simulink model "test_mdl1"  (R2023a)
settings: Solver=VariableStepAuto  StartTime=0.0  StopTime=10.0  RelTol=1e-3
(part 4 of 8)

== system test_mdl1/VehicleCAN/GWM/Climate_Cntrl_Data_2_FD1 ==
  AutoStpHvacDelta_I_Est : Constant  Value=0
  CabnAmb_Te_Actl : Constant  Value=0
  ClimtThrmlLoad_No_Actl : Constant  Value=0
  HvacAir_Flw_Est : Constant  Value=0
  HvacBlwrFront_D_Stat : Constant  Value=0
  HvacRec_Pc_Est : Constant  Value=0
  HvacRemoteStrt_N_Rq : Constant  Value=0
  bus_creator : BusCreator  Inputs=7
  out_port : Outport
  wires:
  bus_creator/1 -> out_port/1  "test_mdl1"
  AutoStpHvacDelta_I_Est/1 -> bus_creator/1  "AutoStpHvacDelta_I_Est"
  CabnAmb_Te_Actl/1 -> bus_creator/2  "CabnAmb_Te_Actl"
  ClimtThrmlLoad_No_Actl/1 -> bus_creator/3  "ClimtThrmlLoad_No_Actl"
  HvacAir_Flw_Est/1 -> bus_creator/4  "HvacAir_Flw_Est"
  HvacBlwrFront_D_Stat/1 -> bus_creator/5  "HvacBlwrFront_D_Stat"
  HvacRec_Pc_Est/1 -> bus_creator/6  "HvacRec_Pc_Est"
  HvacRemoteStrt_N_Rq/1 -> bus_creator/7  "HvacRemoteStrt_N_Rq"

== system test_mdl1/VehicleCAN/GWM/Climate_Control_Data_FD1 ==
  AutoHoldSwtch_D_Stat : Constant  Value=0
  LpdbDfrstRearOn_B_Rq : Constant  Value=0
  LpdbHeatWiprPrk_B_Rq : Constant  Value=0
  LpdbPtc1_B_Rq : Constant  Value=0
  LpdbPtc2_B_Rq : Constant  Value=0
  LpdbPtc3_B_Rq : Constant  Value=0
  MirrorHeatOn_B_Rq : Constant  Value=0
  Outside_Air_Temp_Stat : Constant  Value=0
  Remote_Start_QuietMode : Constant  Value=0
  SteWhlHeat_D_Rq : Constant  Value=0
  bus_creator : BusCreator  Inputs=10
  out_port : Outport
  wires:
  bus_creator/1 -> out_port/1  "test_mdl1"
  AutoHoldSwtch_D_Stat/1 -> bus_creator/1  "AutoHoldSwtch_D_Stat"
  LpdbDfrstRearOn_B_Rq/1 -> bus_creator/2  "LpdbDfrstRearOn_B_Rq"
  LpdbHeatWiprPrk_B_Rq/1 -> bus_creator/3  "LpdbHeatWiprPrk_B_Rq"
  LpdbPtc1_B_Rq/1 -> bus_creator/4  "LpdbPtc1_B_Rq"
  LpdbPtc2_B_Rq/1 -> bus_creator/5  "LpdbPtc2_B_Rq"
  LpdbPtc3_B_Rq/1 -> bus_creator/6  "LpdbPtc3_B_Rq"
  MirrorHeatOn_B_Rq/1 -> bus_creator/7  "MirrorHeatOn_B_Rq"
  Outside_Air_Temp_Stat/1 -> bus_creator/8  "Outside_Air_Temp_Stat"
  Remote_Start_QuietMode/1 -> bus_creator/9  "Remote_Start_QuietMode"
  SteWhlHeat_D_Rq/1 -> bus_creator/10  "SteWhlHeat_D_Rq"

== system test_mdl1/VehicleCAN/GWM/Cluster_HEV_Data8_FD1 ==
  ConsAvgTrip_Fe_Dsply : Constant  Value=0
  DrvEffLvl_No_Stat : Constant  Value=0
  EngAirFilt_B_RqReset : Constant  Value=0
  GpsElMdeSel_B_Rq : Constant  Value=0
  LongTermReset_B_Rq : Constant  Value=0
  bus_creator : BusCreator  Inputs=5
  out_port : Outport
  wires:
  bus_creator/1 -> out_port/1  "test_mdl1"
  ConsAvgTrip_Fe_Dsply/1 -> bus_creator/1  "ConsAvgTrip_Fe_Dsply"
  DrvEffLvl_No_Stat/1 -> bus_creator/2  "DrvEffLvl_No_Stat"
  EngAirFilt_B_RqReset/1 -> bus_creator/3  "EngAirFilt_B_RqReset"
  GpsElMdeSel_B_Rq/1 -> bus_creator/4  "GpsElMdeSel_B_Rq"
  LongTermReset_B_Rq/1 -> bus_creator/5  "LongTermReset_B_Rq"

== system test_mdl1/VehicleCAN/GWM/Cluster_Info1_FD1 ==
  AccDeny_B_RqIpc : Constant  Value=0
  AccEnbl_B_RqDrv : Constant  Value=0
  BulbChkActv_B_Stat : Constant  Value=0
  DrvSlipCtlMde_B_Rq2 : Constant  Value=0
  DrvSlipCtlMde_D_Rq : Constant  Value=0
  EngIdlShutDown_B_RqDrv : Constant  Value=0
  EngOilLife_B_RqReset : Constant  Value=0
  HaDsplyCpblty_B_Stat : Constant  Value=0
  HsaMde_D_Rq : Constant  Value=0
  KeyTypeChngMykey_D_Rq : Constant  Value=0
  LscmbbStat_B_Actl : Constant  Value=0
  ManRgen_D_Rq : Constant  Value=0
  MetricActv_B_Actl : Constant  Value=0
  NtrlTowMdeEnbl_B_RqDrv : Constant  Value=0
  OdometerMasterValue : Constant  Value=0
  ParkDetect_Stat : Constant  Value=0
  Power_Liftgate_Mode_Cmd : Constant  Value=0
  ReducedGuard_D_Rq : Constant  Value=0
  TRAILER_BRAKE_CONFIG : Constant  Value=0
  TRLR_SWAY_CONFIG_CMD : Constant  Value=0
  TrlrBrkMde_D_Rq : Constant  Value=0
  bus_creator : BusCreator  Inputs=22
  ePRNDL_MODE : Constant  Value=0
  out_port : Outport
  wires:
  bus_creator/1 -> out_port/1  "test_mdl1"
  AccDeny_B_RqIpc/1 -> bus_creator/1  "AccDeny_B_RqIpc"
  AccEnbl_B_RqDrv/1 -> bus_creator/2  "AccEnbl_B_RqDrv"
  BulbChkActv_B_Stat/1 -> bus_creator/3  "BulbChkActv_B_Stat"
  DrvSlipCtlMde_B_Rq2/1 -> bus_creator/4  "DrvSlipCtlMde_B_Rq2"
  DrvSlipCtlMde_D_Rq/1 -> bus_creator/5  "DrvSlipCtlMde_D_Rq"
  EngIdlShutDown_B_RqDrv/1 -> bus_creator/6  "EngIdlShutDown_B_RqDrv"
  EngOilLife_B_RqReset/1 -> bus_creator/7  "EngOilLife_B_RqReset"
  HaDsplyCpblty_B_Stat/1 -> bus_creator/8  "HaDsplyCpblty_B_Stat"
  HsaMde_D_Rq/1 -> bus_creator/9  "HsaMde_D_Rq"
  KeyTypeChngMykey_D_Rq/1 -> bus_creator/10  "KeyTypeChngMykey_D_Rq"
  LscmbbStat_B_Actl/1 -> bus_creator/11  "LscmbbStat_B_Actl"
  ManRgen_D_Rq/1 -> bus_creator/12  "ManRgen_D_Rq"
  MetricActv_B_Actl/1 -> bus_creator/13  "MetricActv_B_Actl"
  NtrlTowMdeEnbl_B_RqDrv/1 -> bus_creator/14  "NtrlTowMdeEnbl_B_RqDrv"
  OdometerMasterValue/1 -> bus_creator/15  "OdometerMasterValue"
  ParkDetect_Stat/1 -> bus_creator/16  "ParkDetect_Stat"
  Power_Liftgate_Mode_Cmd/1 -> bus_creator/17  "Power_Liftgate_Mode_Cmd"
  ReducedGuard_D_Rq/1 -> bus_creator/18  "ReducedGuard_D_Rq"
  TRAILER_BRAKE_CONFIG/1 -> bus_creator/19  "TRAILER_BRAKE_CONFIG"
  TRLR_SWAY_CONFIG_CMD/1 -> bus_creator/20  "TRLR_SWAY_CONFIG_CMD"
  TrlrBrkMde_D_Rq/1 -> bus_creator/21  "TrlrBrkMde_D_Rq"
  ePRNDL_MODE/1 -> bus_creator/22  "ePRNDL_MODE"

== system test_mdl1/VehicleCAN/GWM/Cluster_Info_3_FD1 ==
  AutoRgen_D_Rq : Constant  Value=0
  DISPLAY_SPEED_OFFSET : Constant  Value=0
  DISPLAY_SPEED_SCALING : Constant  Value=0
  DrvSlipCtlMde_B_RqMyKey : Constant  Value=0
  FUEL_SENSOR_NUM : Constant  Value=0
  FuelLvlActvSide_No_Raw : Constant  Value=0
  FuelLvlPssvSide_No_Raw : Constant  Value=0
  FuelLvlWarn_D_Actl : Constant  Value=0
  FuelLvl_Pc_Dsply : Constant  Value=0
  FuelSecndActv_B_Actl : Constant  Value=0
  HILL_DESC_SW : Constant  Value=0
  OdoTripRx_B_Actl : Constant  Value=0
  Veh_V_CompLimMx : Constant  Value=0
  W2S_LAMP_OK : Constant  Value=0
  bus_creator : BusCreator  Inputs=14
  out_port : Outport
  wires:
  bus_creator/1 -> out_port/1  "test_mdl1"
  AutoRgen_D_Rq/1 -> bus_creator/1  "AutoRgen_D_Rq"
  DISPLAY_SPEED_OFFSET/1 -> bus_creator/2  "DISPLAY_SPEED_OFFSET"
  DISPLAY_SPEED_SCALING/1 -> bus_creator/3  "DISPLAY_SPEED_SCALING"
  DrvSlipCtlMde_B_RqMyKey/1 -> bus_creator/4  "DrvSlipCtlMde_B_RqMyKey"
  FUEL_SENSOR_NUM/1 -> bus_creator/5  "FUEL_SENSOR_NUM"
  FuelLvlActvSide_No_Raw/1 -> bus_creator/6  "FuelLvlActvSide_No_Raw"
  FuelLvlPssvSide_No_Raw/1 -> bus_creator/7  "FuelLvlPssvSide_No_Raw"
  FuelLvlWarn_D_Actl/1 -> bus_creator/8  "FuelLvlWarn_D_Actl"
  FuelLvl_Pc_Dsply/1 -> bus_creator/9  "FuelLvl_Pc_Dsply"
  FuelSecndActv_B_Actl/1 -> bus_creator/10  "FuelSecndActv_B_Actl"
  HILL_DESC_SW/1 -> bus_creator/11  "HILL_DESC_SW"
  OdoTripRx_B_Actl/1 -> bus_creator/12  "OdoTripRx_B_Actl"
  Veh_V_CompLimMx/1 -> bus_creator/13  "Veh_V_CompLimMx"
  W2S_LAMP_OK/1 -> bus_creator/14  "W2S_LAMP_OK"

== system test_mdl1/VehicleCAN/GWM/Cluster_Lighting_Rq_FD1 ==
  IsaOffst_D_Rq : Constant  Value=0
  SlMde_D_Rq : Constant  Value=0
  bus_creator : BusCreator  Inputs=2
  out_port : Outport
  wires:
  bus_creator/1 -> out_port/1  "test_mdl1"
  IsaOffst_D_Rq/1 -> bus_creator/1  "IsaOffst_D_Rq"
  SlMde_D_Rq/1 -> bus_creator/2  "SlMde_D_Rq"

== system test_mdl1/VehicleCAN/GWM/Compressor_Req_FD1 ==
  ClimtCool_D_Rq : Constant  Value=0
  ClimtHeat_D_Rq : Constant  Value=0
  ClimtPw_B_Rq : Constant  Value=0
  HvacAirCond_B_Rq : Constant  Value=0
  HvacEvap_Te_Actl : Constant  Value=0
  HvacEvap_Te_Offst : Constant  Value=0
  HvacEvap_Te_Rq : Constant  Value=0
  HvacHtrCore_Te_Rq : Constant  Value=0
  SnowPlowMde_B_Enbl : Constant  Value=0
  StopStrtDrvMde_B_RqBtn : Constant  Value=0
  bus_creator : BusCreator  Inputs=10
  out_port : Outport
  wires:
  bus_creator/1 -> out_port/1  "test_mdl1"
  ClimtCool_D_Rq/1 -> bus_creator/1  "ClimtCool_D_Rq"
  ClimtHeat_D_Rq/1 -> bus_creator/2  "ClimtHeat_D_Rq"
  ClimtPw_B_Rq/1 -> bus_creator/3  "ClimtPw_B_Rq"
  HvacAirCond_B_Rq/1 -> bus_creator/4  "HvacAirCond_B_Rq"
  HvacEvap_Te_Actl/1 -> bus_creator/5  "HvacEvap_Te_Actl"
  HvacEvap_Te_Offst/1 -> bus_creator/6  "HvacEvap_Te_Offst"
  HvacEvap_Te_Rq/1 -> bus_creator/7  "HvacEvap_Te_Rq"
  HvacHtrCore_Te_Rq/1 -> bus_creator/8  "HvacHtrCore_Te_Rq"
  SnowPlowMde_B_Enbl/1 -> bus_creator/9  "SnowPlowMde_B_Enbl"
  StopStrtDrvMde_B_RqBtn/1 -> bus_creator/10  "StopStrtDrvMde_B_RqBtn"

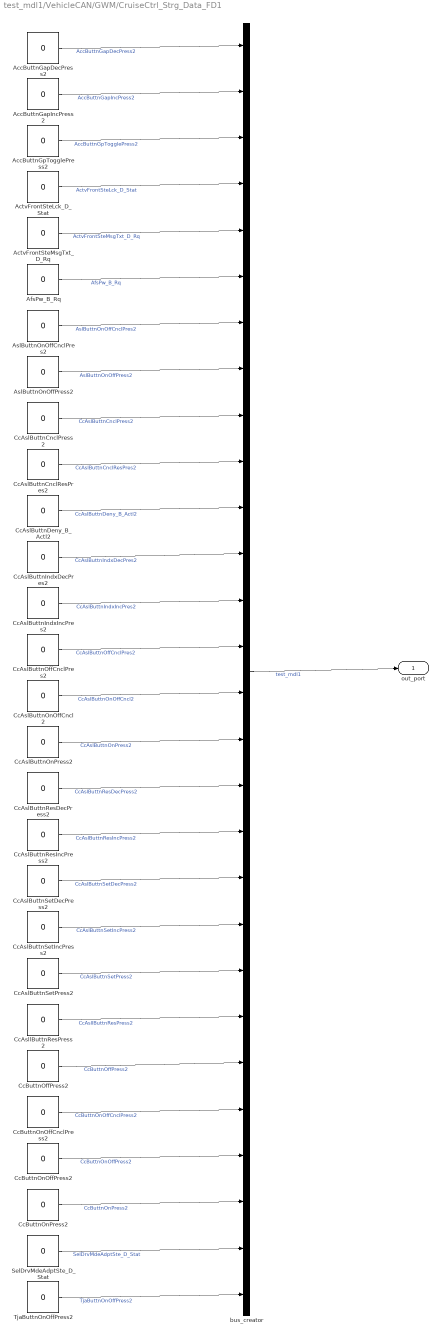
== system test_mdl1/VehicleCAN/GWM/CruiseCtrl_Strg_Data_FD1 ==
  AccButtnGapDecPress2 : Constant  Value=0
  AccButtnGapIncPress2 : Constant  Value=0
  AccButtnGpTogglePress2 : Constant  Value=0
  ActvFrontSteLck_D_Stat : Constant  Value=0
  ActvFrontSteMsgTxt_D_Rq : Constant  Value=0
  AfsPw_B_Rq : Constant  Value=0
  AslButtnOnOffCnclPres2 : Constant  Value=0
  AslButtnOnOffPress2 : Constant  Value=0
  CcAslButtnCnclPress2 : Constant  Value=0
  CcAslButtnCnclResPres2 : Constant  Value=0
  CcAslButtnDeny_B_Actl2 : Constant  Value=0
  CcAslButtnIndxDecPres2 : Constant  Value=0
  CcAslButtnIndxIncPres2 : Constant  Value=0
  CcAslButtnOffCnclPres2 : Constant  Value=0
  CcAslButtnOnOffCncl2 : Constant  Value=0
  CcAslButtnOnPress2 : Constant  Value=0
  CcAslButtnResDecPress2 : Constant  Value=0
  CcAslButtnResIncPress2 : Constant  Value=0
  CcAslButtnSetDecPress2 : Constant  Value=0
  CcAslButtnSetIncPress2 : Constant  Value=0
  CcAslButtnSetPress2 : Constant  Value=0
  CcAsllButtnResPress2 : Constant  Value=0
  CcButtnOffPress2 : Constant  Value=0
  CcButtnOnOffCnclPress2 : Constant  Value=0
  CcButtnOnOffPress2 : Constant  Value=0
  CcButtnOnPress2 : Constant  Value=0
  SelDrvMdeAdptSte_D_Stat : Constant  Value=0
  TjaButtnOnOffPress2 : Constant  Value=0
  bus_creator : BusCreator  Inputs=28
  out_port : Outport
  wires:
  bus_creator/1 -> out_port/1  "test_mdl1"
  AccButtnGapDecPress2/1 -> bus_creator/1  "AccButtnGapDecPress2"
  AccButtnGapIncPress2/1 -> bus_creator/2  "AccButtnGapIncPress2"
  AccButtnGpTogglePress2/1 -> bus_creator/3  "AccButtnGpTogglePress2"
  ActvFrontSteLck_D_Stat/1 -> bus_creator/4  "ActvFrontSteLck_D_Stat"
  ActvFrontSteMsgTxt_D_Rq/1 -> bus_creator/5  "ActvFrontSteMsgTxt_D_Rq"
  AfsPw_B_Rq/1 -> bus_creator/6  "AfsPw_B_Rq"
  AslButtnOnOffCnclPres2/1 -> bus_creator/7  "AslButtnOnOffCnclPres2"
  AslButtnOnOffPress2/1 -> bus_creator/8  "AslButtnOnOffPress2"
  CcAslButtnCnclPress2/1 -> bus_creator/9  "CcAslButtnCnclPress2"
  CcAslButtnCnclResPres2/1 -> bus_creator/10  "CcAslButtnCnclResPres2"
  CcAslButtnDeny_B_Actl2/1 -> bus_creator/11  "CcAslButtnDeny_B_Actl2"
  CcAslButtnIndxDecPres2/1 -> bus_creator/12  "CcAslButtnIndxDecPres2"
  CcAslButtnIndxIncPres2/1 -> bus_creator/13  "CcAslButtnIndxIncPres2"
  CcAslButtnOffCnclPres2/1 -> bus_creator/14  "CcAslButtnOffCnclPres2"
  CcAslButtnOnOffCncl2/1 -> bus_creator/15  "CcAslButtnOnOffCncl2"
  CcAslButtnOnPress2/1 -> bus_creator/16  "CcAslButtnOnPress2"
  CcAslButtnResDecPress2/1 -> bus_creator/17  "CcAslButtnResDecPress2"
  CcAslButtnResIncPress2/1 -> bus_creator/18  "CcAslButtnResIncPress2"
  CcAslButtnSetDecPress2/1 -> bus_creator/19  "CcAslButtnSetDecPress2"
  CcAslButtnSetIncPress2/1 -> bus_creator/20  "CcAslButtnSetIncPress2"
  CcAslButtnSetPress2/1 -> bus_creator/21  "CcAslButtnSetPress2"
  CcAsllButtnResPress2/1 -> bus_creator/22  "CcAsllButtnResPress2"
  CcButtnOffPress2/1 -> bus_creator/23  "CcButtnOffPress2"
  CcButtnOnOffCnclPress2/1 -> bus_creator/24  "CcButtnOnOffCnclPress2"
  CcButtnOnOffPress2/1 -> bus_creator/25  "CcButtnOnOffPress2"
  CcButtnOnPress2/1 -> bus_creator/26  "CcButtnOnPress2"
  SelDrvMdeAdptSte_D_Stat/1 -> bus_creator/27  "SelDrvMdeAdptSte_D_Stat"
  TjaButtnOnOffPress2/1 -> bus_creator/28  "TjaButtnOnOffPress2"

== system test_mdl1/VehicleCAN/GWM/DCACA_Data1_FD1 ==
  CoolFanDcac_D_Rq : Constant  Value=0
  DcacAcUDetct_B_Falt : Constant  Value=0
  DcacBp1BrkrOpn_B_Falt : Constant  Value=0
  DcacBp2BrkrOpn_B_Falt : Constant  Value=0
  DcacClntFlw_D_Rq : Constant  Value=0
  DcacErr_B_Stat : Constant  Value=0
  DcacGfci_B_Falt : Constant  Value=0
  DcacIpRcBrkrOpn_B_Falt : Constant  Value=0
  DcacOverTe_B_Falt : Constant  Value=0
  DcacOvrld_B_Falt : Constant  Value=0
  DcacPlugPrsnt_B_Stat : Constant  Value=0
  DcacRdy_D2_Stat : Constant  Value=0
  DcacRdy_D_Stat : Constant  Value=0
  bus_creator : BusCreator  Inputs=13
  out_port : Outport
  wires:
  bus_creator/1 -> out_port/1  "test_mdl1"
  CoolFanDcac_D_Rq/1 -> bus_creator/1  "CoolFanDcac_D_Rq"
  DcacAcUDetct_B_Falt/1 -> bus_creator/2  "DcacAcUDetct_B_Falt"
  DcacBp1BrkrOpn_B_Falt/1 -> bus_creator/3  "DcacBp1BrkrOpn_B_Falt"
  DcacBp2BrkrOpn_B_Falt/1 -> bus_creator/4  "DcacBp2BrkrOpn_B_Falt"
  DcacClntFlw_D_Rq/1 -> bus_creator/5  "DcacClntFlw_D_Rq"
  DcacErr_B_Stat/1 -> bus_creator/6  "DcacErr_B_Stat"
  DcacGfci_B_Falt/1 -> bus_creator/7  "DcacGfci_B_Falt"
  DcacIpRcBrkrOpn_B_Falt/1 -> bus_creator/8  "DcacIpRcBrkrOpn_B_Falt"
  DcacOverTe_B_Falt/1 -> bus_creator/9  "DcacOverTe_B_Falt"
  DcacOvrld_B_Falt/1 -> bus_creator/10  "DcacOvrld_B_Falt"
  DcacPlugPrsnt_B_Stat/1 -> bus_creator/11  "DcacPlugPrsnt_B_Stat"
  DcacRdy_D2_Stat/1 -> bus_creator/12  "DcacRdy_D2_Stat"
  DcacRdy_D_Stat/1 -> bus_creator/13  "DcacRdy_D_Stat"

== system test_mdl1/VehicleCAN/GWM/DCACA_Data2_FD1 ==
  DcacIn_I_Actl : Constant  Value=0
  DcacIn_U2_Actl : Constant  Value=0
  DcacIn_U_Actl : Constant  Value=0
  Dcac_Te_Actl : Constant  Value=0
  bus_creator : BusCreator  Inputs=4
  out_port : Outport
  wires:
  bus_creator/1 -> out_port/1  "test_mdl1"
  DcacIn_I_Actl/1 -> bus_creator/1  "DcacIn_I_Actl"
  DcacIn_U2_Actl/1 -> bus_creator/2  "DcacIn_U2_Actl"
  DcacIn_U_Actl/1 -> bus_creator/3  "DcacIn_U_Actl"
  Dcac_Te_Actl/1 -> bus_creator/4  "Dcac_Te_Actl"

== system test_mdl1/VehicleCAN/GWM/DCACA_Data3_FD1 ==
  DcacIn_Pw_Mx : Constant  Value=0
  DcacOut1_Pw_Actl : Constant  Value=0
  DcacOut2_Pw_Actl : Constant  Value=0
  DcacOut_Pw_Mx : Constant  Value=0
  bus_creator : BusCreator  Inputs=4
  out_port : Outport
  wires:
  bus_creator/1 -> out_port/1  "test_mdl1"
  DcacIn_Pw_Mx/1 -> bus_creator/1  "DcacIn_Pw_Mx"
  DcacOut1_Pw_Actl/1 -> bus_creator/2  "DcacOut1_Pw_Actl"
  DcacOut2_Pw_Actl/1 -> bus_creator/3  "DcacOut2_Pw_Actl"
  DcacOut_Pw_Mx/1 -> bus_creator/4  "DcacOut_Pw_Mx"

== system test_mdl1/VehicleCAN/GWM/DTE_ECGtoHPCM ==
  DteCldBattULo_Eff_Actl : Constant  Value=0
  DteCldClimt_Eff_Actl : Constant  Value=0
  DteCldDcac_B_Stat : Constant  Value=0
  DteCldDrv_Eff_Actl : Constant  Value=0
  DteCldExtTe_B_Stat : Constant  Value=0
  DteCldExt_Eff_Actl : Constant  Value=0
  DteCldId_No_Actl : Constant  Value=0
  DteCldPayload_B_Stat : Constant  Value=0
  DteCldRoute_B_Stat : Constant  Value=0
  DteCldTerrain_B_Stat : Constant  Value=0
  DteCldTraffic_B_Stat : Constant  Value=0
  DteCldTrip_L_Actl : Constant  Value=0
  DteCldTrlrOff_B_Stat : Constant  Value=0
  DteCldTrlrOn_B_Stat : Constant  Value=0
  bus_creator : BusCreator  Inputs=14
  out_port : Outport
  wires:
  bus_creator/1 -> out_port/1  "test_mdl1"
  DteCldBattULo_Eff_Actl/1 -> bus_creator/1  "DteCldBattULo_Eff_Actl"
  DteCldClimt_Eff_Actl/1 -> bus_creator/2  "DteCldClimt_Eff_Actl"
  DteCldDcac_B_Stat/1 -> bus_creator/3  "DteCldDcac_B_Stat"
  DteCldDrv_Eff_Actl/1 -> bus_creator/4  "DteCldDrv_Eff_Actl"
  DteCldExtTe_B_Stat/1 -> bus_creator/5  "DteCldExtTe_B_Stat"
  DteCldExt_Eff_Actl/1 -> bus_creator/6  "DteCldExt_Eff_Actl"
  DteCldId_No_Actl/1 -> bus_creator/7  "DteCldId_No_Actl"
  DteCldPayload_B_Stat/1 -> bus_creator/8  "DteCldPayload_B_Stat"
  DteCldRoute_B_Stat/1 -> bus_creator/9  "DteCldRoute_B_Stat"
  DteCldTerrain_B_Stat/1 -> bus_creator/10  "DteCldTerrain_B_Stat"
  DteCldTraffic_B_Stat/1 -> bus_creator/11  "DteCldTraffic_B_Stat"
  DteCldTrip_L_Actl/1 -> bus_creator/12  "DteCldTrip_L_Actl"
  DteCldTrlrOff_B_Stat/1 -> bus_creator/13  "DteCldTrlrOff_B_Stat"
  DteCldTrlrOn_B_Stat/1 -> bus_creator/14  "DteCldTrlrOn_B_Stat"

== system test_mdl1/VehicleCAN/GWM/Driver_Dr_Stat_FD1 ==
  BLISLEDStatDriverSide : Constant  Value=0
  ChildLckFdbckRd_B_Stat : Constant  Value=0
  ChildLckPw_D_Rq : Constant  Value=0
  ChildLckPw_N_Cnt : Constant  Value=0
  Driver_Lock_Sw_Cnt : Constant  Value=0
  Driver_Lock_Sw_Stat : Constant  Value=0
  KeyCylSwDrvDr_D_Stat : Constant  Value=0
  RollCodeDrvDrKeyCyl : Constant  Value=0
  RvrseMirrorChime_B_Rq : Constant  Value=0
  WndwDrvSide_D_Stat : Constant  Value=0
  bus_creator : BusCreator  Inputs=10
  out_port : Outport
  wires:
  bus_creator/1 -> out_port/1  "test_mdl1"
  BLISLEDStatDriverSide/1 -> bus_creator/1  "BLISLEDStatDriverSide"
  ChildLckFdbckRd_B_Stat/1 -> bus_creator/2  "ChildLckFdbckRd_B_Stat"
  ChildLckPw_D_Rq/1 -> bus_creator/3  "ChildLckPw_D_Rq"
  ChildLckPw_N_Cnt/1 -> bus_creator/4  "ChildLckPw_N_Cnt"
  Driver_Lock_Sw_Cnt/1 -> bus_creator/5  "Driver_Lock_Sw_Cnt"
  Driver_Lock_Sw_Stat/1 -> bus_creator/6  "Driver_Lock_Sw_Stat"
  KeyCylSwDrvDr_D_Stat/1 -> bus_creator/7  "KeyCylSwDrvDr_D_Stat"
  RollCodeDrvDrKeyCyl/1 -> bus_creator/8  "RollCodeDrvDrKeyCyl"
  RvrseMirrorChime_B_Rq/1 -> bus_creator/9  "RvrseMirrorChime_B_Rq"
  WndwDrvSide_D_Stat/1 -> bus_creator/10  "WndwDrvSide_D_Stat"

== system test_mdl1/VehicleCAN/GWM/Dsp_Request_Signals11_FD1 ==
  ApaMdeStat_D_RqDrv : Constant  Value=0
  ApaSwtch_D_RqMnu : Constant  Value=0
  CamAutoTowbarZoom : Constant  Value=0
  CamraOvrlDyn_D_Rq : Constant  Value=0
  CamraOvrlStat_D_Rq : Constant  Value=0
  CamraViewSplit_B_Rq : Constant  Value=0
  CamraZoomMan_D_Rq : Constant  Value=0
  DistanceBarSetting : Constant  Value=0
  PrkAidSwtch_D_RqMnu : Constant  Value=0
  bus_creator : BusCreator  Inputs=9
  out_port : Outport
  wires:
  bus_creator/1 -> out_port/1  "test_mdl1"
  ApaMdeStat_D_RqDrv/1 -> bus_creator/1  "ApaMdeStat_D_RqDrv"
  ApaSwtch_D_RqMnu/1 -> bus_creator/2  "ApaSwtch_D_RqMnu"
  CamAutoTowbarZoom/1 -> bus_creator/3  "CamAutoTowbarZoom"
  CamraOvrlDyn_D_Rq/1 -> bus_creator/4  "CamraOvrlDyn_D_Rq"
  CamraOvrlStat_D_Rq/1 -> bus_creator/5  "CamraOvrlStat_D_Rq"
  CamraViewSplit_B_Rq/1 -> bus_creator/6  "CamraViewSplit_B_Rq"
  CamraZoomMan_D_Rq/1 -> bus_creator/7  "CamraZoomMan_D_Rq"
  DistanceBarSetting/1 -> bus_creator/8  "DistanceBarSetting"
  PrkAidSwtch_D_RqMnu/1 -> bus_creator/9  "PrkAidSwtch_D_RqMnu"

== system test_mdl1/VehicleCAN/GWM/ECG_Data2_FD1 ==
  DataMntrSustn_B_Rq : Constant  Value=0
  DgtlCommPncReset_B_Req : Constant  Value=0
  PwSustnRdata_B_RqTelem : Constant  Value=0
  bus_creator : BusCreator  Inputs=3
  out_port : Outport
  wires:
  bus_creator/1 -> out_port/1  "test_mdl1"
  DataMntrSustn_B_Rq/1 -> bus_creator/1  "DataMntrSustn_B_Rq"
  DgtlCommPncReset_B_Req/1 -> bus_creator/2  "DgtlCommPncReset_B_Req"
  PwSustnRdata_B_RqTelem/1 -> bus_creator/3  "PwSustnRdata_B_RqTelem"

== system test_mdl1/VehicleCAN/GWM/ECG_Data3_FD1 ==
  BattULoChrg_D_RqOta : Constant  Value=0
  CanMsg375_No_Cnt : Constant  Value=0
  CanMsg375_No_Crc : Constant  Value=0
  OtaActv_D_Stat : Constant  Value=0
  VehOnRqstr_D_Stat : Constant  Value=0
  VehOn_D_RqCld : Constant  Value=0
  VehStrtInhbt_D_Dsply : Constant  Value=0
  VehStrtInhbt_D_RqCld : Constant  Value=0
  VehStrtInhbt_T_Dsply : Constant  Value=0
  bus_creator : BusCreator  Inputs=9
  out_port : Outport
  wires:
  bus_creator/1 -> out_port/1  "test_mdl1"
  BattULoChrg_D_RqOta/1 -> bus_creator/1  "BattULoChrg_D_RqOta"
  CanMsg375_No_Cnt/1 -> bus_creator/2  "CanMsg375_No_Cnt"
  CanMsg375_No_Crc/1 -> bus_creator/3  "CanMsg375_No_Crc"
  OtaActv_D_Stat/1 -> bus_creator/4  "OtaActv_D_Stat"
  VehOnRqstr_D_Stat/1 -> bus_creator/5  "VehOnRqstr_D_Stat"
  VehOn_D_RqCld/1 -> bus_creator/6  "VehOn_D_RqCld"
  VehStrtInhbt_D_Dsply/1 -> bus_creator/7  "VehStrtInhbt_D_Dsply"
  VehStrtInhbt_D_RqCld/1 -> bus_creator/8  "VehStrtInhbt_D_RqCld"
  VehStrtInhbt_T_Dsply/1 -> bus_creator/9  "VehStrtInhbt_T_Dsply"

== system test_mdl1/VehicleCAN/GWM/ECG_Data4_FD1 ==
  PtWakeupActv1_B_Rq : Constant  Value=0
  bus_creator : BusCreator  Inputs=1
  out_port : Outport
  wires:
  bus_creator/1 -> out_port/1  "test_mdl1"
  PtWakeupActv1_B_Rq/1 -> bus_creator/1  "PtWakeupActv1_B_Rq"

== system test_mdl1/VehicleCAN/GWM/ECG_Data_FD1 ==
  ChrgrPncEnbl_D_Rq : Constant  Value=0
  ChrgrPncSustn_B_Rq : Constant  Value=0
  ExtLghtDsply_B_StatArb : Constant  Value=0
  ExtLghtFront_D_RqOta : Constant  Value=0
  ExtLghtLeft_D_RqOta : Constant  Value=0
  ExtLghtRear_D_RqOta : Constant  Value=0
  ExtLghtRight_D_RqOta : Constant  Value=0
  NtfyDrvSocLvl1_Pc_Rq : Constant  Value=0
  NtfyDrvTrgtDist_L_Rq : Constant  Value=0
  OBCCSerial_D_Rq : Constant  Value=0
  PtRmtRprt_D_Stat : Constant  Value=0
  TlghtTest_D_RqArb : Constant  Value=0
  bus_creator : BusCreator  Inputs=12
  out_port : Outport
  wires:
  bus_creator/1 -> out_port/1  "test_mdl1"
  ChrgrPncEnbl_D_Rq/1 -> bus_creator/1  "ChrgrPncEnbl_D_Rq"
  ChrgrPncSustn_B_Rq/1 -> bus_creator/2  "ChrgrPncSustn_B_Rq"
  ExtLghtDsply_B_StatArb/1 -> bus_creator/3  "ExtLghtDsply_B_StatArb"
  ExtLghtFront_D_RqOta/1 -> bus_creator/4  "ExtLghtFront_D_RqOta"
  ExtLghtLeft_D_RqOta/1 -> bus_creator/5  "ExtLghtLeft_D_RqOta"
  ExtLghtRear_D_RqOta/1 -> bus_creator/6  "ExtLghtRear_D_RqOta"
  ExtLghtRight_D_RqOta/1 -> bus_creator/7  "ExtLghtRight_D_RqOta"
  NtfyDrvSocLvl1_Pc_Rq/1 -> bus_creator/8  "NtfyDrvSocLvl1_Pc_Rq"
  NtfyDrvTrgtDist_L_Rq/1 -> bus_creator/9  "NtfyDrvTrgtDist_L_Rq"
  OBCCSerial_D_Rq/1 -> bus_creator/10  "OBCCSerial_D_Rq"
  PtRmtRprt_D_Stat/1 -> bus_creator/11  "PtRmtRprt_D_Stat"
  TlghtTest_D_RqArb/1 -> bus_creator/12  "TlghtTest_D_RqArb"

== system test_mdl1/VehicleCAN/GWM/ElecHorizon_Data1_FD1 ==
  EhData1_No_Actl : Constant  Value=0
  bus_creator : BusCreator  Inputs=1
  out_port : Outport
  wires:
  bus_creator/1 -> out_port/1  "test_mdl1"
  EhData1_No_Actl/1 -> bus_creator/1  "EhData1_No_Actl"

== system test_mdl1/VehicleCAN/GWM/ElecHorizon_Data2_FD1 ==
  EhData2_No_Actl : Constant  Value=0
  bus_creator : BusCreator  Inputs=1
  out_port : Outport
  wires:
  bus_creator/1 -> out_port/1  "test_mdl1"
  EhData2_No_Actl/1 -> bus_creator/1  "EhData2_No_Actl"

== system test_mdl1/VehicleCAN/GWM/FourByFourSwitchData_FD1 ==
  AwdMde_D_RqDrv : Constant  Value=0
  DrvSlipCtlMde_B_Rq3 : Constant  Value=0
  HdcSwtchPos_B_Actl : Constant  Value=0
  HybMdeSwtch_B_Rq : Constant  Value=0
  RearDiffLck_D_RqDrv : Constant  Value=0
  TrailCtlSwtch_B_Stat3 : Constant  Value=0
  bus_creator : BusCreator  Inputs=6
  out_port : Outport
  wires:
  bus_creator/1 -> out_port/1  "test_mdl1"
  AwdMde_D_RqDrv/1 -> bus_creator/1  "AwdMde_D_RqDrv"
  DrvSlipCtlMde_B_Rq3/1 -> bus_creator/2  "DrvSlipCtlMde_B_Rq3"
  HdcSwtchPos_B_Actl/1 -> bus_creator/3  "HdcSwtchPos_B_Actl"
  HybMdeSwtch_B_Rq/1 -> bus_creator/4  "HybMdeSwtch_B_Rq"
  RearDiffLck_D_RqDrv/1 -> bus_creator/5  "RearDiffLck_D_RqDrv"
  TrailCtlSwtch_B_Stat3/1 -> bus_creator/6  "TrailCtlSwtch_B_Stat3"

== system test_mdl1/VehicleCAN/GWM/GGCC_Config_Mgmt_ID_1_FD1 ==
  VehicleGGCCData : Constant  Value=0
  bus_creator : BusCreator  Inputs=1
  out_port : Outport
  wires:
  bus_creator/1 -> out_port/1  "test_mdl1"
  VehicleGGCCData/1 -> bus_creator/1  "VehicleGGCCData"

== system test_mdl1/VehicleCAN/GWM/GWM_AutoSar_NetMgmt_FD1 ==
  GWM_AutoSarNMControl : Constant  Value=0
  GWM_AutoSarNMNodeId : Constant  Value=0
  GWM_AutoSarNMReserved{1..4} (4 alike) : Constant  Value=0
  GWM_GWNMProxy : Constant  Value=0
  GWM_GWOnBoardTester : Constant  Value=0
  bus_creator : BusCreator  Inputs=8
  out_port : Outport
  wires:
  bus_creator/1 -> out_port/1  "test_mdl1"
  GWM_AutoSarNMControl/1 -> bus_creator/1  "GWM_AutoSarNMControl"
  GWM_AutoSarNMNodeId/1 -> bus_creator/2  "GWM_AutoSarNMNodeId"
  GWM_AutoSarNMReserved1/1 -> bus_creator/3  "GWM_AutoSarNMReserved1"
  GWM_AutoSarNMReserved2/1 -> bus_creator/4  "GWM_AutoSarNMReserved2"
  GWM_AutoSarNMReserved3/1 -> bus_creator/5  "GWM_AutoSarNMReserved3"
  GWM_AutoSarNMReserved4/1 -> bus_creator/6  "GWM_AutoSarNMReserved4"
  GWM_GWNMProxy/1 -> bus_creator/7  "GWM_GWNMProxy"
  GWM_GWOnBoardTester/1 -> bus_creator/8  "GWM_GWOnBoardTester"

== system test_mdl1/VehicleCAN/GWM/Gear_Shift_by_Wire_2_FD1 ==
  GearButtnStuck_B_Actl : Constant  Value=0
  GsmSrvcRqd_B_Rq : Constant  Value=0
  TrnGearPwmFalt_B_Actl : Constant  Value=0
  bus_creator : BusCreator  Inputs=3
  out_port : Outport
  wires:
  bus_creator/1 -> out_port/1  "test_mdl1"
  GearButtnStuck_B_Actl/1 -> bus_creator/1  "GearButtnStuck_B_Actl"
  GsmSrvcRqd_B_Rq/1 -> bus_creator/2  "GsmSrvcRqd_B_Rq"
  TrnGearPwmFalt_B_Actl/1 -> bus_creator/3  "TrnGearPwmFalt_B_Actl"

== system test_mdl1/VehicleCAN/GWM/Gear_Shift_by_Wire_FD1 ==
  BrkSwtchPos_B_ActlGsm : Constant  Value=0
  DrQltyDrv_D_StatGsm : Constant  Value=0
  GsmGearMsgTxt_D_Rq : Constant  Value=0
  PrkBrkActv_D_RqGsmGear : Constant  Value=0
  TrnBtsiOvrrd_B_Stat : Constant  Value=0
  TrnGearButtn_B_ActlD0 : Constant  Value=0
  TrnGearButtn_B_ActlD1 : Constant  Value=0
  TrnGearButtn_B_ActlD2 : Constant  Value=0
  TrnGearButtn_B_ActlM0 : Constant  Value=0
  TrnGearButtn_B_ActlM1 : Constant  Value=0
  TrnGearButtn_B_ActlM2 : Constant  Value=0
  TrnGearButtn_B_ActlN0 : Constant  Value=0
  TrnGearButtn_B_ActlN1 : Constant  Value=0
  TrnGearButtn_B_ActlN2 : Constant  Value=0
  TrnGearButtn_B_ActlP0 : Constant  Value=0
  TrnGearButtn_B_ActlP1 : Constant  Value=0
  TrnGearButtn_B_ActlP2 : Constant  Value=0
  TrnGearButtn_B_ActlR0 : Constant  Value=0
  TrnGearButtn_B_ActlR1 : Constant  Value=0
  TrnGearButtn_B_ActlR2 : Constant  Value=0
  TrnGearButtn_U_Actl : Constant  Value=0
  TrnGearRqCnt_B_Actl : Constant  Value=0
  TrnGear_D_RqDrv : Constant  Value=0
  TrnGear_No_Cnt : Constant  Value=0
  TrnGear_No_Cs : Constant  Value=0
  TrnGsmNtmState_D_Actl : Constant  Value=0
  TrnRng_D_RqGsm : Constant  Value=0
  TrnValidGearRq_D_Stat : Constant  Value=0
  bus_creator : BusCreator  Inputs=28
  out_port : Outport
  wires:
  bus_creator/1 -> out_port/1  "test_mdl1"
  BrkSwtchPos_B_ActlGsm/1 -> bus_creator/1  "BrkSwtchPos_B_ActlGsm"
  DrQltyDrv_D_StatGsm/1 -> bus_creator/2  "DrQltyDrv_D_StatGsm"
  GsmGearMsgTxt_D_Rq/1 -> bus_creator/3  "GsmGearMsgTxt_D_Rq"
  PrkBrkActv_D_RqGsmGear/1 -> bus_creator/4  "PrkBrkActv_D_RqGsmGear"
  TrnBtsiOvrrd_B_Stat/1 -> bus_creator/5  "TrnBtsiOvrrd_B_Stat"
  TrnGearButtn_B_ActlD0/1 -> bus_creator/6  "TrnGearButtn_B_ActlD0"
  TrnGearButtn_B_ActlD1/1 -> bus_creator/7  "TrnGearButtn_B_ActlD1"
  TrnGearButtn_B_ActlD2/1 -> bus_creator/8  "TrnGearButtn_B_ActlD2"
  TrnGearButtn_B_ActlM0/1 -> bus_creator/9  "TrnGearButtn_B_ActlM0"
  TrnGearButtn_B_ActlM1/1 -> bus_creator/10  "TrnGearButtn_B_ActlM1"
  TrnGearButtn_B_ActlM2/1 -> bus_creator/11  "TrnGearButtn_B_ActlM2"
  TrnGearButtn_B_ActlN0/1 -> bus_creator/12  "TrnGearButtn_B_ActlN0"
  TrnGearButtn_B_ActlN1/1 -> bus_creator/13  "TrnGearButtn_B_ActlN1"
  TrnGearButtn_B_ActlN2/1 -> bus_creator/14  "TrnGearButtn_B_ActlN2"
  TrnGearButtn_B_ActlP0/1 -> bus_creator/15  "TrnGearButtn_B_ActlP0"
  TrnGearButtn_B_ActlP1/1 -> bus_creator/16  "TrnGearButtn_B_ActlP1"
  TrnGearButtn_B_ActlP2/1 -> bus_creator/17  "TrnGearButtn_B_ActlP2"
  TrnGearButtn_B_ActlR0/1 -> bus_creator/18  "TrnGearButtn_B_ActlR0"
  TrnGearButtn_B_ActlR1/1 -> bus_creator/19  "TrnGearButtn_B_ActlR1"
  TrnGearButtn_B_ActlR2/1 -> bus_creator/20  "TrnGearButtn_B_ActlR2"
  TrnGearButtn_U_Actl/1 -> bus_creator/21  "TrnGearButtn_U_Actl"
  TrnGearRqCnt_B_Actl/1 -> bus_creator/22  "TrnGearRqCnt_B_Actl"
  TrnGear_D_RqDrv/1 -> bus_creator/23  "TrnGear_D_RqDrv"
  TrnGear_No_Cnt/1 -> bus_creator/24  "TrnGear_No_Cnt"
  TrnGear_No_Cs/1 -> bus_creator/25  "TrnGear_No_Cs"
  TrnGsmNtmState_D_Actl/1 -> bus_creator/26  "TrnGsmNtmState_D_Actl"
  TrnRng_D_RqGsm/1 -> bus_creator/27  "TrnRng_D_RqGsm"
  TrnValidGearRq_D_Stat/1 -> bus_creator/28  "TrnValidGearRq_D_Stat"

== system test_mdl1/VehicleCAN/GWM/GlobalClock_Data_FD1 ==
  GlblClkDay_No_Actl : Constant  Value=0
  GlblClkHr_No_Actl : Constant  Value=0
  GlblClkMnte_No_Actl : Constant  Value=0
  GlblClkScnd_No_Actl : Constant  Value=0
  GlblClkYr_No_Actl : Constant  Value=0
  bus_creator : BusCreator  Inputs=5
  out_port : Outport
  wires:
  bus_creator/1 -> out_port/1  "test_mdl1"
  GlblClkDay_No_Actl/1 -> bus_creator/1  "GlblClkDay_No_Actl"
  GlblClkHr_No_Actl/1 -> bus_creator/2  "GlblClkHr_No_Actl"
  GlblClkMnte_No_Actl/1 -> bus_creator/3  "GlblClkMnte_No_Actl"
  GlblClkScnd_No_Actl/1 -> bus_creator/4  "GlblClkScnd_No_Actl"
  GlblClkYr_No_Actl/1 -> bus_creator/5  "GlblClkYr_No_Actl"

== system test_mdl1/VehicleCAN/GWM/Global_PATS_Cntrl_Info_FD1 ==
  bus_creator : BusCreator  Inputs=2
  immoControlCmd_T1 : Constant  Value=0
  immoControlData_T1 : Constant  Value=0
  out_port : Outport
  wires:
  bus_creator/1 -> out_port/1  "test_mdl1"
  immoControlCmd_T1/1 -> bus_creator/1  "immoControlCmd_T1"
  immoControlData_T1/1 -> bus_creator/2  "immoControlData_T1"

== system test_mdl1/VehicleCAN/GWM/Global_PATS_Ctrl_Info2_FD1 ==
  bus_creator : BusCreator  Inputs=2
  immoControlCmd_T2 : Constant  Value=0
  immoControlData_T2 : Constant  Value=0
  out_port : Outport
  wires:
  bus_creator/1 -> out_port/1  "test_mdl1"
  immoControlCmd_T2/1 -> bus_creator/1  "immoControlCmd_T2"
  immoControlData_T2/1 -> bus_creator/2  "immoControlData_T2"

== system test_mdl1/VehicleCAN/GWM/HeadUpDisplayReq_FD1 ==
  SelDrvMdeCnfm_D_Stat : Constant  Value=0
  bus_creator : BusCreator  Inputs=1
  out_port : Outport
  wires:
  bus_creator/1 -> out_port/1  "test_mdl1"
  SelDrvMdeCnfm_D_Stat/1 -> bus_creator/1  "SelDrvMdeCnfm_D_Stat"

== system test_mdl1/VehicleCAN/GWM/IPC_Infotainment_FD1 ==
  BeltminderAudioMute : Constant  Value=0
  Chime_Source : Constant  Value=0
  HdcOn_B_Rq : Constant  Value=0
  IPC_Attn_Info_Audio : Constant  Value=0
  IPC_MyKeyVolLimit_St : Constant  Value=0
  IPC_New_Attn_Event : Constant  Value=0
  Power_Up_Chime_Modules : Constant  Value=0
  Veh_V2_Dsply : Constant  Value=0
  bus_creator : BusCreator  Inputs=8
  out_port : Outport
  wires:
  bus_creator/1 -> out_port/1  "test_mdl1"
  BeltminderAudioMute/1 -> bus_creator/1  "BeltminderAudioMute"
  Chime_Source/1 -> bus_creator/2  "Chime_Source"
  HdcOn_B_Rq/1 -> bus_creator/3  "HdcOn_B_Rq"
  IPC_Attn_Info_Audio/1 -> bus_creator/4  "IPC_Attn_Info_Audio"
  IPC_MyKeyVolLimit_St/1 -> bus_creator/5  "IPC_MyKeyVolLimit_St"
  IPC_New_Attn_Event/1 -> bus_creator/6  "IPC_New_Attn_Event"
  Power_Up_Chime_Modules/1 -> bus_creator/7  "Power_Up_Chime_Modules"
  Veh_V2_Dsply/1 -> bus_creator/8  "Veh_V2_Dsply"

== system test_mdl1/VehicleCAN/GWM/IPC_Send_Signals_2_FD1 ==
  ElLongTerm_L_Dsply : Constant  Value=0
  ElTrip_L_Dsply : Constant  Value=0
  FuelRange_L_Dsply : Constant  Value=0
  bus_creator : BusCreator  Inputs=3
  out_port : Outport
  wires:
  bus_creator/1 -> out_port/1  "test_mdl1"
  ElLongTerm_L_Dsply/1 -> bus_creator/1  "ElLongTerm_L_Dsply"
  ElTrip_L_Dsply/1 -> bus_creator/2  "ElTrip_L_Dsply"
  FuelRange_L_Dsply/1 -> bus_creator/3  "FuelRange_L_Dsply"

== system test_mdl1/VehicleCAN/GWM/LocationServices_3_FD1 ==
  LocationServices_3 : Constant  Value=0
  bus_creator : BusCreator  Inputs=1
  out_port : Outport
  wires:
  bus_creator/1 -> out_port/1  "test_mdl1"
  LocationServices_3/1 -> bus_creator/1  "LocationServices_3"

== system test_mdl1/VehicleCAN/GWM/LocationServices_Data1_FD1 ==
  LocationServices_1 : Constant  Value=0
  bus_creator : BusCreator  Inputs=1
  out_port : Outport
  wires:
  bus_creator/1 -> out_port/1  "test_mdl1"
  LocationServices_1/1 -> bus_creator/1  "LocationServices_1"

== system test_mdl1/VehicleCAN/GWM/Locking_Systems_2_FD1 ==
  ChildLckMde_B_Stat : Constant  Value=0
  ChildLck_D_Dsply : Constant  Value=0
  DrTgateExtSwMde_B_Stat : Constant  Value=0
  DrTgateOpen_B_Rq : Constant  Value=0
  FobComm_D_Stat : Constant  Value=0
  Keyfob_Pad_Msg_Count : Constant  Value=0
  L_Pwr_Sliding_Dr_Rqst : Constant  Value=0
  LockInhibit : Constant  Value=0
  Lockmsgtxt_D_Rq : Constant  Value=0
  Power_Decklid_Rqst : Constant  Value=0
  Power_Liftgate_Rqst : Constant  Value=0
  R_Pwr_Sliding_Dr_Rqst : Constant  Value=0
  Remote_Device_Feedback : Constant  Value=0
  RollCodeUnlock : Constant  Value=0
  VehLckInd_D_Rq : Constant  Value=0
  Veh_Lock_EvNum : Constant  Value=0
  Veh_Lock_Requestor : Constant  Value=0
  Veh_Lock_Status : Constant  Value=0
  Veh_Lock_Sub_Id : Constant  Value=0
  WindowLockout_B_Stat : Constant  Value=0
  bus_creator : BusCreator  Inputs=20
  out_port : Outport
  wires:
  bus_creator/1 -> out_port/1  "test_mdl1"
  ChildLckMde_B_Stat/1 -> bus_creator/1  "ChildLckMde_B_Stat"
  ChildLck_D_Dsply/1 -> bus_creator/2  "ChildLck_D_Dsply"
  DrTgateExtSwMde_B_Stat/1 -> bus_creator/3  "DrTgateExtSwMde_B_Stat"
  DrTgateOpen_B_Rq/1 -> bus_creator/4  "DrTgateOpen_B_Rq"
  FobComm_D_Stat/1 -> bus_creator/5  "FobComm_D_Stat"
  Keyfob_Pad_Msg_Count/1 -> bus_creator/6  "Keyfob_Pad_Msg_Count"
  L_Pwr_Sliding_Dr_Rqst/1 -> bus_creator/7  "L_Pwr_Sliding_Dr_Rqst"
  LockInhibit/1 -> bus_creator/8  "LockInhibit"
  Lockmsgtxt_D_Rq/1 -> bus_creator/9  "Lockmsgtxt_D_Rq"
  Power_Decklid_Rqst/1 -> bus_creator/10  "Power_Decklid_Rqst"
  Power_Liftgate_Rqst/1 -> bus_creator/11  "Power_Liftgate_Rqst"
  R_Pwr_Sliding_Dr_Rqst/1 -> bus_creator/12  "R_Pwr_Sliding_Dr_Rqst"
  Remote_Device_Feedback/1 -> bus_creator/13  "Remote_Device_Feedback"
  RollCodeUnlock/1 -> bus_creator/14  "RollCodeUnlock"
  VehLckInd_D_Rq/1 -> bus_creator/15  "VehLckInd_D_Rq"
  Veh_Lock_EvNum/1 -> bus_creator/16  "Veh_Lock_EvNum"
  Veh_Lock_Requestor/1 -> bus_creator/17  "Veh_Lock_Requestor"
  Veh_Lock_Status/1 -> bus_creator/18  "Veh_Lock_Status"
  Veh_Lock_Sub_Id/1 -> bus_creator/19  "Veh_Lock_Sub_Id"
  WindowLockout_B_Stat/1 -> bus_creator/20  "WindowLockout_B_Stat"

== system test_mdl1/VehicleCAN/GWM/MasterReset_HS3_ECGDat_FD1 ==
  DrvBhavWarn_B_Rq : Constant  Value=0
  FactoryReset_St : Constant  Value=0
  KeyOffPwMde_D_Stat : Constant  Value=0
  ModemReset_D_Stat : Constant  Value=0
  OfbChrgSetSync_D_Rq : Constant  Value=0
  bus_creator : BusCreator  Inputs=5
  out_port : Outport
  wires:
  bus_creator/1 -> out_port/1  "test_mdl1"
  DrvBhavWarn_B_Rq/1 -> bus_creator/1  "DrvBhavWarn_B_Rq"
  FactoryReset_St/1 -> bus_creator/2  "FactoryReset_St"
  KeyOffPwMde_D_Stat/1 -> bus_creator/3  "KeyOffPwMde_D_Stat"
  ModemReset_D_Stat/1 -> bus_creator/4  "ModemReset_D_Stat"
  OfbChrgSetSync_D_Rq/1 -> bus_creator/5  "OfbChrgSetSync_D_Rq"

== system test_mdl1/VehicleCAN/GWM/Mc_Send_Signals_2_FD1 ==
  AwdRnge_D_ActlIpc : Constant  Value=0
  BalrMde_D_Rq : Constant  Value=0
  BalrSwtch_D_Stat : Constant  Value=0
  BttOn_B_Rq : Constant  Value=0
  Btt_L_Actl : Constant  Value=0
  DrvInputRequired_B_Rq : Constant  Value=0
  EdmSailMde_B_RqDrv : Constant  Value=0
  EngExhMdeQuiet_D2_Rq : Constant  Value=0
  EsaOn_B_Rq : Constant  Value=0
  Mc_VehLangUsrSel_St : Constant  Value=0
  Mc_VehTimeFrmtUsrSel_St : Constant  Value=0
  Mc_VehUnitTempUsrSel_St : Constant  Value=0
  Mc_VehUntTrpCoUsrSel_St : Constant  Value=0
  Running_Board_Cmd : Constant  Value=0
  SelDrvMdeDsply_B_Avail : Constant  Value=0
  SelDrvMdeTxtReset_B_Rq : Constant  Value=0
  WaitToStartLamp_D_Falt : Constant  Value=0
  bus_creator : BusCreator  Inputs=17
  out_port : Outport
  wires:
  bus_creator/1 -> out_port/1  "test_mdl1"
  AwdRnge_D_ActlIpc/1 -> bus_creator/1  "AwdRnge_D_ActlIpc"
  BalrMde_D_Rq/1 -> bus_creator/2  "BalrMde_D_Rq"
  BalrSwtch_D_Stat/1 -> bus_creator/3  "BalrSwtch_D_Stat"
  BttOn_B_Rq/1 -> bus_creator/4  "BttOn_B_Rq"
  Btt_L_Actl/1 -> bus_creator/5  "Btt_L_Actl"
  DrvInputRequired_B_Rq/1 -> bus_creator/6  "DrvInputRequired_B_Rq"
  EdmSailMde_B_RqDrv/1 -> bus_creator/7  "EdmSailMde_B_RqDrv"
  EngExhMdeQuiet_D2_Rq/1 -> bus_creator/8  "EngExhMdeQuiet_D2_Rq"
  EsaOn_B_Rq/1 -> bus_creator/9  "EsaOn_B_Rq"
  Mc_VehLangUsrSel_St/1 -> bus_creator/10  "Mc_VehLangUsrSel_St"
  Mc_VehTimeFrmtUsrSel_St/1 -> bus_creator/11  "Mc_VehTimeFrmtUsrSel_St"
  Mc_VehUnitTempUsrSel_St/1 -> bus_creator/12  "Mc_VehUnitTempUsrSel_St"
  Mc_VehUntTrpCoUsrSel_St/1 -> bus_creator/13  "Mc_VehUntTrpCoUsrSel_St"
  Running_Board_Cmd/1 -> bus_creator/14  "Running_Board_Cmd"
  SelDrvMdeDsply_B_Avail/1 -> bus_creator/15  "SelDrvMdeDsply_B_Avail"
  SelDrvMdeTxtReset_B_Rq/1 -> bus_creator/16  "SelDrvMdeTxtReset_B_Rq"
  WaitToStartLamp_D_Falt/1 -> bus_creator/17  "WaitToStartLamp_D_Falt"

== system test_mdl1/VehicleCAN/GWM/OTAFuncGWM_ECG_FD1 ==
  OTAFuncGWM_ECG : Constant  Value=0
  bus_creator : BusCreator  Inputs=1
  out_port : Outport
  wires:
  bus_creator/1 -> out_port/1  "test_mdl1"
  OTAFuncGWM_ECG/1 -> bus_creator/1  "OTAFuncGWM_ECG"

== system test_mdl1/VehicleCAN/GWM/OTAPhysGWM_ECGtoABS ==
  OTAPhysGWM_ECGtoABS : Constant  Value=0
  bus_creator : BusCreator  Inputs=1
  out_port : Outport
  wires:
  bus_creator/1 -> out_port/1  "test_mdl1"
  OTAPhysGWM_ECGtoABS/1 -> bus_creator/1  "OTAPhysGWM_ECGtoABS"

== system test_mdl1/VehicleCAN/GWM/OTAPhysGWM_ECGtoCCM ==
  OTAPhysGWM_ECGtoCCM : Constant  Value=0
  bus_creator : BusCreator  Inputs=1
  out_port : Outport
  wires:
  bus_creator/1 -> out_port/1  "test_mdl1"
  OTAPhysGWM_ECGtoCCM/1 -> bus_creator/1  "OTAPhysGWM_ECGtoCCM"

== system test_mdl1/VehicleCAN/GWM/OTAPhysGWM_ECGtoIPMA ==
  OTAPhysGWM_ECGtoIPMA : Constant  Value=0
  bus_creator : BusCreator  Inputs=1
  out_port : Outport
  wires:
  bus_creator/1 -> out_port/1  "test_mdl1"
  OTAPhysGWM_ECGtoIPMA/1 -> bus_creator/1  "OTAPhysGWM_ECGtoIPMA"

== system test_mdl1/VehicleCAN/GWM/OTAPhysGWM_ECGtoPCM ==
  OTAPhysGWM_ECGtoPCM : Constant  Value=0
  bus_creator : BusCreator  Inputs=1
  out_port : Outport
  wires:
  bus_creator/1 -> out_port/1  "test_mdl1"
  OTAPhysGWM_ECGtoPCM/1 -> bus_creator/1  "OTAPhysGWM_ECGtoPCM"

== system test_mdl1/VehicleCAN/GWM/OTAPhysGWM_ECGtoSOBDMC_FD1 ==
  OTAPhysGWM_ECGtoHPCM : Constant  Value=0
  bus_creator : BusCreator  Inputs=1
  out_port : Outport
  wires:
  bus_creator/1 -> out_port/1  "test_mdl1"
  OTAPhysGWM_ECGtoHPCM/1 -> bus_creator/1  "OTAPhysGWM_ECGtoHPCM"

== system test_mdl1/VehicleCAN/GWM/OTAPhysGWM_ECGtoSODCMC ==
  OTAPhysGWM_ECGtoSODCMC : Constant  Value=0
  bus_creator : BusCreator  Inputs=1
  out_port : Outport
  wires:
  bus_creator/1 -> out_port/1  "test_mdl1"
  OTAPhysGWM_ECGtoSODCMC/1 -> bus_creator/1  "OTAPhysGWM_ECGtoSODCMC"

== system test_mdl1/VehicleCAN/GWM/OTAPhysGWM_ECGtoSODCMD ==
  OTAPhysGWM_ECGtoSODCMD : Constant  Value=0
  bus_creator : BusCreator  Inputs=1
  out_port : Outport
  wires:
  bus_creator/1 -> out_port/1  "test_mdl1"
  OTAPhysGWM_ECGtoSODCMD/1 -> bus_creator/1  "OTAPhysGWM_ECGtoSODCMD"

== system test_mdl1/VehicleCAN/GWM/OTAPhysGWM_ECGtoSODL ==
  OTAPhysGWM_ECGtoSODL : Constant  Value=0
  bus_creator : BusCreator  Inputs=1
  out_port : Outport
  wires:
  bus_creator/1 -> out_port/1  "test_mdl1"
  OTAPhysGWM_ECGtoSODL/1 -> bus_creator/1  "OTAPhysGWM_ECGtoSODL"

== system test_mdl1/VehicleCAN/GWM/OTAPhysGWM_ECGtoSODR ==
  OTAPhysGWM_ECGtoSODR : Constant  Value=0
  bus_creator : BusCreator  Inputs=1
  out_port : Outport
  wires:
  bus_creator/1 -> out_port/1  "test_mdl1"
  OTAPhysGWM_ECGtoSODR/1 -> bus_creator/1  "OTAPhysGWM_ECGtoSODR"

== system test_mdl1/VehicleCAN/GWM/OffBrdChrg_Signals ==
  OfbChrgLocIdTrgt_No_Rq : Constant  Value=0
  OfbChrgLocIdUns_B_Rq : Constant  Value=0
  OfbChrgPrflWkdy_No_Rq : Constant  Value=0
  OfbChrgPrflWknd_No_Rq : Constant  Value=0
  OfbChrgSetDelete_B_Rq : Constant  Value=0
  OfbChrgSetNow_D_Rq : Constant  Value=0
  OfbChrgToPcWkdy_D_Actl : Constant  Value=0
  OfbChrgToPcWknd_D_Actl : Constant  Value=0
  bus_creator : BusCreator  Inputs=8
  out_port : Outport
  wires:
  bus_creator/1 -> out_port/1  "test_mdl1"
  OfbChrgLocIdTrgt_No_Rq/1 -> bus_creator/1  "OfbChrgLocIdTrgt_No_Rq"
  OfbChrgLocIdUns_B_Rq/1 -> bus_creator/2  "OfbChrgLocIdUns_B_Rq"
  OfbChrgPrflWkdy_No_Rq/1 -> bus_creator/3  "OfbChrgPrflWkdy_No_Rq"
  OfbChrgPrflWknd_No_Rq/1 -> bus_creator/4  "OfbChrgPrflWknd_No_Rq"
  OfbChrgSetDelete_B_Rq/1 -> bus_creator/5  "OfbChrgSetDelete_B_Rq"
  OfbChrgSetNow_D_Rq/1 -> bus_creator/6  "OfbChrgSetNow_D_Rq"
  OfbChrgToPcWkdy_D_Actl/1 -> bus_creator/7  "OfbChrgToPcWkdy_D_Actl"
  OfbChrgToPcWknd_D_Actl/1 -> bus_creator/8  "OfbChrgToPcWknd_D_Actl"

== system test_mdl1/VehicleCAN/GWM/OffBrdChrg_Signals2 ==
  OfbChrgClearAll_B_Rq : Constant  Value=0
  OfbChrgGoTDelete_B_Rq : Constant  Value=0
  OfbChrgGoTElement_D_Rq : Constant  Value=0
  OfbChrgGoTExtHtr_D_Rq : Constant  Value=0
  OfbChrgGoTHr_T_Rq : Constant  Value=0
  OfbChrgGoTMnte_D_Rq : Constant  Value=0
  OfbChrgGoTOn_D_Rq : Constant  Value=0
  OfbChrgGoTPrcond_D_Rq : Constant  Value=0
  OfbChrgGoTTouch_D_Rq : Constant  Value=0
  OfbChrgGoTUpdate_B_Rq : Constant  Value=0
  OfbChrgPrflUpdate_B_Rq : Constant  Value=0
  bus_creator : BusCreator  Inputs=11
  out_port : Outport
  wires:
  bus_creator/1 -> out_port/1  "test_mdl1"
  OfbChrgClearAll_B_Rq/1 -> bus_creator/1  "OfbChrgClearAll_B_Rq"
  OfbChrgGoTDelete_B_Rq/1 -> bus_creator/2  "OfbChrgGoTDelete_B_Rq"
  OfbChrgGoTElement_D_Rq/1 -> bus_creator/3  "OfbChrgGoTElement_D_Rq"
  OfbChrgGoTExtHtr_D_Rq/1 -> bus_creator/4  "OfbChrgGoTExtHtr_D_Rq"
  OfbChrgGoTHr_T_Rq/1 -> bus_creator/5  "OfbChrgGoTHr_T_Rq"
  OfbChrgGoTMnte_D_Rq/1 -> bus_creator/6  "OfbChrgGoTMnte_D_Rq"
  OfbChrgGoTOn_D_Rq/1 -> bus_creator/7  "OfbChrgGoTOn_D_Rq"
  OfbChrgGoTPrcond_D_Rq/1 -> bus_creator/8  "OfbChrgGoTPrcond_D_Rq"
  OfbChrgGoTTouch_D_Rq/1 -> bus_creator/9  "OfbChrgGoTTouch_D_Rq"
  OfbChrgGoTUpdate_B_Rq/1 -> bus_creator/10  "OfbChrgGoTUpdate_B_Rq"
  OfbChrgPrflUpdate_B_Rq/1 -> bus_creator/11  "OfbChrgPrflUpdate_B_Rq"

== system test_mdl1/VehicleCAN/GWM/PARSEDFuncGWM_ECG_FD1 ==
  PARSEDFuncGWM_ECG : Constant  Value=0
  bus_creator : BusCreator  Inputs=1
  out_port : Outport
  wires:
  bus_creator/1 -> out_port/1  "test_mdl1"
  PARSEDFuncGWM_ECG/1 -> bus_creator/1  "PARSEDFuncGWM_ECG"

== system test_mdl1/VehicleCAN/GWM/PARSEDPhysGWM_ECGtoABS ==
  PARSEDPhysGWM_ECGtoABS : Constant  Value=0
  bus_creator : BusCreator  Inputs=1
  out_port : Outport
  wires:
  bus_creator/1 -> out_port/1  "test_mdl1"
  PARSEDPhysGWM_ECGtoABS/1 -> bus_creator/1  "PARSEDPhysGWM_ECGtoABS"

== system test_mdl1/VehicleCAN/GWM/PARSEDPhysGWM_ECGtoCCM ==
  PARSEDPhysGWM_ECGtoCCM : Constant  Value=0
  bus_creator : BusCreator  Inputs=1
  out_port : Outport
  wires:
  bus_creator/1 -> out_port/1  "test_mdl1"
  PARSEDPhysGWM_ECGtoCCM/1 -> bus_creator/1  "PARSEDPhysGWM_ECGtoCCM"

== system test_mdl1/VehicleCAN/GWM/PARSEDPhysGWM_ECGtoIPMA ==
  PARSEDPhysGWM_ECGtoIPMA : Constant  Value=0
  bus_creator : BusCreator  Inputs=1
  out_port : Outport
  wires:
  bus_creator/1 -> out_port/1  "test_mdl1"
  PARSEDPhysGWM_ECGtoIPMA/1 -> bus_creator/1  "PARSEDPhysGWM_ECGtoIPMA"

== system test_mdl1/VehicleCAN/GWM/PARSEDPhysGWM_ECGtoPCM ==
  PARSEDPhysGWM_ECGtoPCM : Constant  Value=0
  bus_creator : BusCreator  Inputs=1
  out_port : Outport
  wires:
  bus_creator/1 -> out_port/1  "test_mdl1"
  PARSEDPhysGWM_ECGtoPCM/1 -> bus_creator/1  "PARSEDPhysGWM_ECGtoPCM"

== system test_mdl1/VehicleCAN/GWM/PARSEDPhysGWM_ECGtoSODCMC ==
  PARSEDPhysGWM_ECGtoSODCMC : Constant  Value=0
  bus_creator : BusCreator  Inputs=1
  out_port : Outport
  wires:
  bus_creator/1 -> out_port/1  "test_mdl1"
  PARSEDPhysGWM_ECGtoSODCMC/1 -> bus_creator/1  "PARSEDPhysGWM_ECGtoSODCMC"

== system test_mdl1/VehicleCAN/GWM/PARSEDPhysGWM_ECGtoSODCMD ==
  PARSEDPhysGWM_ECGtoSODCMD : Constant  Value=0
  bus_creator : BusCreator  Inputs=1
  out_port : Outport
  wires:
  bus_creator/1 -> out_port/1  "test_mdl1"
  PARSEDPhysGWM_ECGtoSODCMD/1 -> bus_creator/1  "PARSEDPhysGWM_ECGtoSODCMD"

== system test_mdl1/VehicleCAN/GWM/PARSEDPhysGWM_ECGtoSODL ==
  PARSEDPhysGWM_ECGtoSODL : Constant  Value=0
  bus_creator : BusCreator  Inputs=1
  out_port : Outport
  wires:
  bus_creator/1 -> out_port/1  "test_mdl1"
  PARSEDPhysGWM_ECGtoSODL/1 -> bus_creator/1  "PARSEDPhysGWM_ECGtoSODL"

== system test_mdl1/VehicleCAN/GWM/PARSEDPhysGWM_ECGtoSODR ==
  PARSEDPhysGWM_ECGtoSODR : Constant  Value=0
  bus_creator : BusCreator  Inputs=1
  out_port : Outport
  wires:
  bus_creator/1 -> out_port/1  "test_mdl1"
  PARSEDPhysGWM_ECGtoSODR/1 -> bus_creator/1  "PARSEDPhysGWM_ECGtoSODR"

== system test_mdl1/VehicleCAN/GWM/PARSEDPhysGWMtoSOBDMC_FD1 ==
  PARSEDPhysGWM_ECGtoHPCM : Constant  Value=0
  bus_creator : BusCreator  Inputs=1
  out_port : Outport
  wires:
  bus_creator/1 -> out_port/1  "test_mdl1"
  PARSEDPhysGWM_ECGtoHPCM/1 -> bus_creator/1  "PARSEDPhysGWM_ECGtoHPCM"

== system test_mdl1/VehicleCAN/GWM/PARSEDPushFcGWM_ECGtoABS ==
  PARSEDPhysGWM_ECG2toABS : Constant  Value=0
  bus_creator : BusCreator  Inputs=1
  out_port : Outport
  wires:
  bus_creator/1 -> out_port/1  "test_mdl1"
  PARSEDPhysGWM_ECG2toABS/1 -> bus_creator/1  "PARSEDPhysGWM_ECG2toABS"

== system test_mdl1/VehicleCAN/GWM/PARSEDPushFcGWM_ECGtoPCM ==
  PARSEDPhysGWM_ECG2toPCM : Constant  Value=0
  bus_creator : BusCreator  Inputs=1
  out_port : Outport
  wires:
  bus_creator/1 -> out_port/1  "test_mdl1"
  PARSEDPhysGWM_ECG2toPCM/1 -> bus_creator/1  "PARSEDPhysGWM_ECG2toPCM"

== system test_mdl1/VehicleCAN/GWM/PHEV_Battery_Data1_FD1 ==
  BattAuxCnnct_B_Cmd : Constant  Value=0
  bus_creator : BusCreator  Inputs=1
  out_port : Outport
  wires:
  bus_creator/1 -> out_port/1  "test_mdl1"
  BattAuxCnnct_B_Cmd/1 -> bus_creator/1  "BattAuxCnnct_B_Cmd"

== system test_mdl1/VehicleCAN/GWM/ParkAid_Aud_Warn_CmdM_FD1 ==
  Cta_D_Rq : Constant  Value=0
  PrkAidAcsyFront_D_RqDrv : Constant  Value=0
  PrkAidAcsyRear_D_RqDrv : Constant  Value=0
  PrkAidFront_D_RqDrv : Constant  Value=0
  PrkAidRear_D_RqDrv : Constant  Value=0
  Sod_D_Rq : Constant  Value=0
  SteEffort_D_Rq : Constant  Value=0
  bus_creator : BusCreator  Inputs=7
  out_port : Outport
  wires:
  bus_creator/1 -> out_port/1  "test_mdl1"
  Cta_D_Rq/1 -> bus_creator/1  "Cta_D_Rq"
  PrkAidAcsyFront_D_RqDrv/1 -> bus_creator/2  "PrkAidAcsyFront_D_RqDrv"
  PrkAidAcsyRear_D_RqDrv/1 -> bus_creator/3  "PrkAidAcsyRear_D_RqDrv"
  PrkAidFront_D_RqDrv/1 -> bus_creator/4  "PrkAidFront_D_RqDrv"
  PrkAidRear_D_RqDrv/1 -> bus_creator/5  "PrkAidRear_D_RqDrv"
  Sod_D_Rq/1 -> bus_creator/6  "Sod_D_Rq"
  SteEffort_D_Rq/1 -> bus_creator/7  "SteEffort_D_Rq"

== system test_mdl1/VehicleCAN/GWM/Pass_Dr_Stat_FD1 ==
  BLISLEDStatPassSide : Constant  Value=0
  ChildLckFdbckRp_B_Stat : Constant  Value=0
  Memory_1_SwPsngr_Stat : Constant  Value=0
  Memory_2_SwPsngr_Stat : Constant  Value=0
  Memory_3_SwPsngr_Stat : Constant  Value=0
  Pasngr_Lock_Sw_Cnt : Constant  Value=0
  Pasngr_Lock_Sw_Stat : Constant  Value=0
  RollCode_No_ActlPdm : Constant  Value=0
  WndwPsngrSide_D_Stat : Constant  Value=0
  bus_creator : BusCreator  Inputs=9
  out_port : Outport
  wires:
  bus_creator/1 -> out_port/1  "test_mdl1"
  BLISLEDStatPassSide/1 -> bus_creator/1  "BLISLEDStatPassSide"
  ChildLckFdbckRp_B_Stat/1 -> bus_creator/2  "ChildLckFdbckRp_B_Stat"
  Memory_1_SwPsngr_Stat/1 -> bus_creator/3  "Memory_1_SwPsngr_Stat"
  Memory_2_SwPsngr_Stat/1 -> bus_creator/4  "Memory_2_SwPsngr_Stat"
  Memory_3_SwPsngr_Stat/1 -> bus_creator/5  "Memory_3_SwPsngr_Stat"
  Pasngr_Lock_Sw_Cnt/1 -> bus_creator/6  "Pasngr_Lock_Sw_Cnt"
  Pasngr_Lock_Sw_Stat/1 -> bus_creator/7  "Pasngr_Lock_Sw_Stat"
  RollCode_No_ActlPdm/1 -> bus_creator/8  "RollCode_No_ActlPdm"
  WndwPsngrSide_D_Stat/1 -> bus_creator/9  "WndwPsngrSide_D_Stat"

== system test_mdl1/VehicleCAN/GWM/PowerDistData_2_FD1 ==
  AirCondCluBatt_D_Falt : Constant  Value=0
  AirCondCluGnd_D_Falt : Constant  Value=0
  AirCondCluLife_D_Falt : Constant  Value=0
  AirCondCluOpen_D_Falt : Constant  Value=0
  AirCondClu_D_Stat : Constant  Value=0
  BattChlrLifeLim_D_Falt : Constant  Value=0
  BattChlrOpnCirct_D_Falt : Constant  Value=0
  BattChlrShrtBatt_D_Falt : Constant  Value=0
  BattChlrShrtGrnd_D_Falt : Constant  Value=0
  BattTracLifeLim_D_Falt : Constant  Value=0
  BattTracLow_D_Falt : Constant  Value=0
  BattTracOpnCirct_D_Falt : Constant  Value=0
  BattTracShrtBatt_D_Falt : Constant  Value=0
  BattTracShrtGrnd_D_Falt : Constant  Value=0
  bus_creator : BusCreator  Inputs=14
  out_port : Outport
  wires:
  bus_creator/1 -> out_port/1  "test_mdl1"
  AirCondCluBatt_D_Falt/1 -> bus_creator/1  "AirCondCluBatt_D_Falt"
  AirCondCluGnd_D_Falt/1 -> bus_creator/2  "AirCondCluGnd_D_Falt"
  AirCondCluLife_D_Falt/1 -> bus_creator/3  "AirCondCluLife_D_Falt"
  AirCondCluOpen_D_Falt/1 -> bus_creator/4  "AirCondCluOpen_D_Falt"
  AirCondClu_D_Stat/1 -> bus_creator/5  "AirCondClu_D_Stat"
  BattChlrLifeLim_D_Falt/1 -> bus_creator/6  "BattChlrLifeLim_D_Falt"
  BattChlrOpnCirct_D_Falt/1 -> bus_creator/7  "BattChlrOpnCirct_D_Falt"
  BattChlrShrtBatt_D_Falt/1 -> bus_creator/8  "BattChlrShrtBatt_D_Falt"
  BattChlrShrtGrnd_D_Falt/1 -> bus_creator/9  "BattChlrShrtGrnd_D_Falt"
  BattTracLifeLim_D_Falt/1 -> bus_creator/10  "BattTracLifeLim_D_Falt"
  BattTracLow_D_Falt/1 -> bus_creator/11  "BattTracLow_D_Falt"
  BattTracOpnCirct_D_Falt/1 -> bus_creator/12  "BattTracOpnCirct_D_Falt"
  BattTracShrtBatt_D_Falt/1 -> bus_creator/13  "BattTracShrtBatt_D_Falt"
  BattTracShrtGrnd_D_Falt/1 -> bus_creator/14  "BattTracShrtGrnd_D_Falt"

== system test_mdl1/VehicleCAN/GWM/PowerDist_Data1_FD1 ==
  BattChlrSov_D_Stat : Constant  Value=0
  BattTracClntVlv_D_Stat : Constant  Value=0
  CabnEvapSovFront_D_Stat : Constant  Value=0
  bus_creator : BusCreator  Inputs=3
  out_port : Outport
  wires:
  bus_creator/1 -> out_port/1  "test_mdl1"
  BattChlrSov_D_Stat/1 -> bus_creator/1  "BattChlrSov_D_Stat"
  BattTracClntVlv_D_Stat/1 -> bus_creator/2  "BattTracClntVlv_D_Stat"
  CabnEvapSovFront_D_Stat/1 -> bus_creator/3  "CabnEvapSovFront_D_Stat"
